simulink model "Aircraft_Pitch17"  (R2017a)
settings: Solver=FixedStepAuto  StartTime=0.0  StopTime=30  FixedStep=0.01  RelTol=1e-3
libraries: simulink x1
settings Model: Creator=nikhil  LastModifiedBy=nikhil

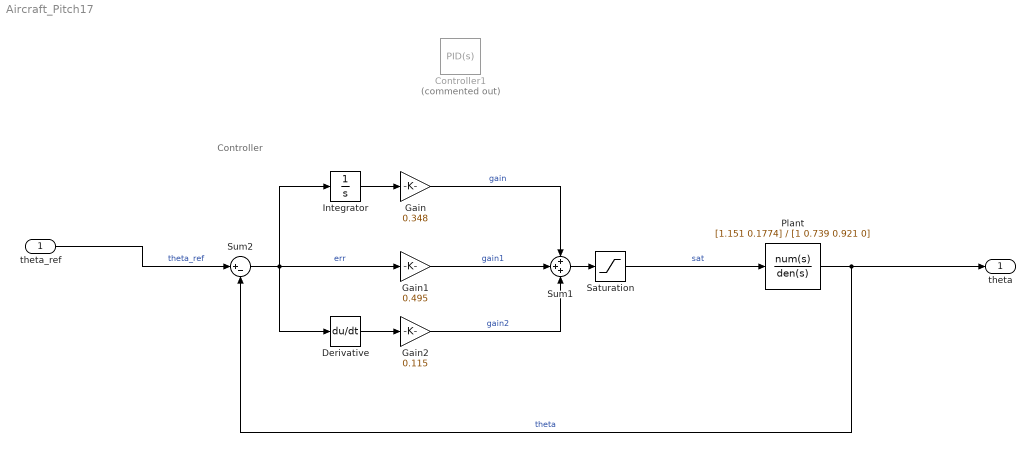
== system Aircraft_Pitch17 ==
  note: Controller
  theta_ref : Inport
  Controller1 : simulink/Continuous/PID Controller  Commented=on  Controller=PID  Form=Parallel  TimeDomain=Continuous-time  SampleTime=-1  IntegratorMethod=Forward Euler  FilterMethod=Forward Euler  ControllerParametersSource=internal  P=0.495489431295944  I=0.348673810814314  D=0.115802581405706  UseFilter=on  N=101.801208075095  InitialConditionSource=internal  InitialConditionForIntegrator=0  InitialConditionForFilter=0  DifferentiatorICPrevScaledInput=0  ExternalReset=none  TrackingMode=off  Kt=1  LimitOutput=off  UpperSaturationLimit=inf  LowerSaturationLimit=-inf  LinearizeAsGain=on  AntiWindupMode=none  Kb=1  POutMin=[]  POutMax=[]  IOutMin=[]  IOutMax=[]  DOutMin=[]  DOutMax=[]  NOutMin=[]  NOutMax=[]  SumOutMin=[]  SumOutMax=[]  SaturationOutMin=[]  SaturationOutMax=[]  PParamMin=[]  PParamMax=[]  IParamMin=[]  IParamMax=[]  DParamMin=[]  DParamMax=[]  NParamMin=[]  NParamMax=[]  KbParamMin=[]  KbParamMax=[]  KtParamMin=[]  KtParamMax=[]  KbOutMin=[]  KbOutMax=[]  KtOutMin=[]  KtOutMax=[]  IntegratorOutMin=[]  IntegratorOutMax=[]  FilterOutMin=[]  FilterOutMax=[]  SumI1OutMin=[]  SumI1OutMax=[]  SumI2OutMin=[]  SumI2OutMax=[]  SumI3OutMin=[]  SumI3OutMax=[]  SumDOutMin=[]  SumDOutMax=[]  DifferentiatorOutMin=[]  DifferentiatorOutMax=[]  IntegratorContinuousStateAttributes=''  IntegratorStateMustResolveToSignalObject=off  IntegratorRTWStateStorageClass=Auto  FilterContinuousStateAttributes=''  FilterStateMustResolveToSignalObject=off  FilterRTWStateStorageClass=Auto
  Derivative : Derivative
  Gain : Gain  Gain=0.348
  Gain1 : Gain  Gain=0.495
  Gain2 : Gain  Gain=0.115
  Integrator : Integrator
  Plant : TransferFcn  Numerator=[1.151 0.1774]  Denominator=[1 0.739 0.921 0]
  Saturation : Saturate  UpperLimit=15  LowerLimit=-15
  Sum1 : Sum  Inputs=+++
  Sum2 : Sum  Inputs=|+-
  theta : Outport
  wires:
  theta_ref/1 -> Sum2/1  "theta_ref"
  Plant/1 -> theta/1, Sum2/2  "theta"
  Gain1/1 -> Sum1/2  "gain1"
  Sum1/1 -> Saturation/1
  Derivative/1 -> Gain2/1
  Sum2/1 -> Derivative/1, Gain1/1, Integrator/1  "err"
  Integrator/1 -> Gain/1
  Gain2/1 -> Sum1/3  "gain2"
  Gain/1 -> Sum1/1  "gain"
  Saturation/1 -> Plant/1  "sat"
